simulink model "punto2"  (R2020b)
settings: Solver=VariableStepAuto  StartTime=0.0  StopTime=10.0  RelTol=1e-3
settings Model: Creator=Acer  LastModifiedBy=Acer

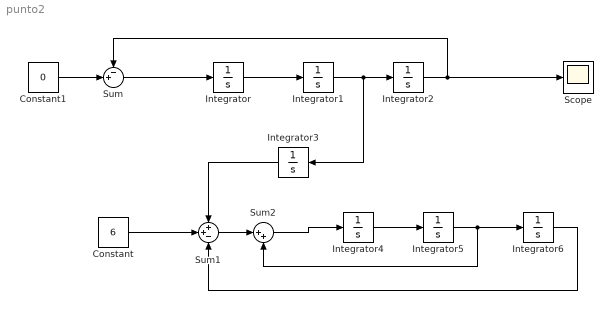
== system punto2 ==
  Constant : Constant  Value=6
  Constant1 : Constant  Value=0
  Integrator{,1..6} (7 alike) : Integrator
  Scope : Scope
  Sum : Sum  Inputs=-+|
  Sum1 : Sum  Inputs=++-
  Sum2 : Sum  Inputs=|++
  wires:
  Integrator/1 -> Integrator1/1
  Integrator1/1 -> Integrator3/1, Integrator2/1
  Sum/1 -> Integrator/1
  Integrator2/1 -> Scope/1, Sum/1
  Integrator3/1 -> Sum1/1
  Constant/1 -> Sum1/2
  Constant1/1 -> Sum/2
  Integrator4/1 -> Integrator5/1
  Sum1/1 -> Sum2/1
  Sum2/1 -> Integrator4/1
  Integrator5/1 -> Integrator6/1, Sum2/2
  Integrator6/1 -> Sum1/3
